simulink model "sunsensor_validity_and_logic_test"  (R2018b)
settings: Solver=VariableStepAuto  StartTime=0.0  StopTime=10.0  RelTol=1e-3
undefined symbols (not defined in the file): simParams
libraries: CDH_command_lib x1, mode_select_lib x1, sunsensor_processing_lib x1
settings Model: Creator=Taylor  LastModifiedBy=Taylor

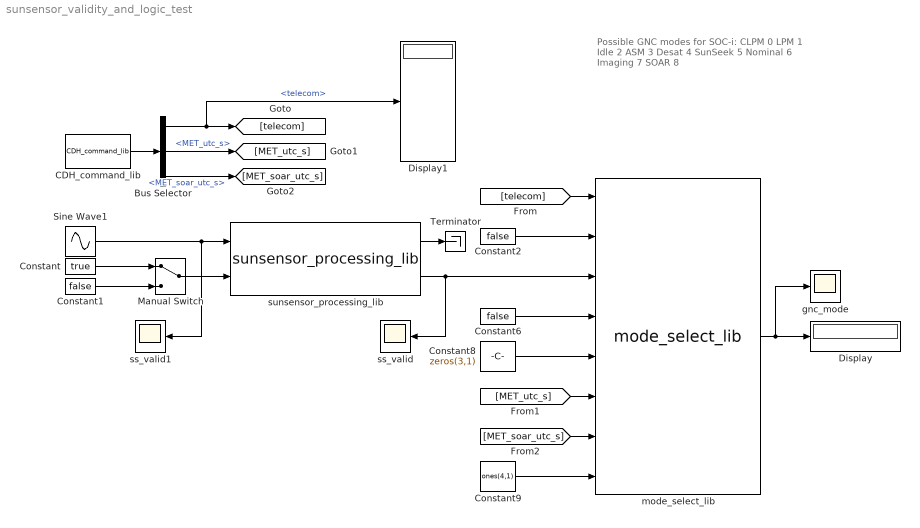
== system sunsensor_validity_and_logic_test ==
  note: Possible GNC modes for SOC-i:
      | CLPM 0
      | LPM 1
      | Idle 2
      | ASM 3
      | Desat 4
      | SunSeek 5
      | Nominal 6
      | Imaging 7
      | SOAR 8
  Bus Selector : BusSelector  OutputSignals=telecom,MET_utc_s,MET_soar_utc_s
  CDH_command_lib : CDH_command_lib/CDH_command_lib  target_lat_deg=47  target_lon_deg=-122  target_alt_m=44  override_autonomy=0  enable_pointing=on  force_clpm=off  force_lpm=off  enable_img=off  enable_soar=off  triad_override=off  MET_soar_utc_s=simParams.time.epoch_utc_s+2000  quat_soar_cmd=[1;0;0;0]
  Constant : Constant  Value=true
  Constant1 : Constant  Value=false
  Constant2 : Constant  Value=false
  Constant6 : Constant  Value=false
  Constant8 : Constant  Value=zeros(3,1)
  Constant9 : Constant  Value=ones(4,1)
  Display : Display
  Display1 : Display
  Manual Switch : ManualSwitch
  Sine Wave1 : Sin  Amplitude=[90 90]  Bias=[0 0]  Frequency=[1 1]  Phase=[0 0]  SampleTime=0
  Terminator : Terminator
  gnc_mode : Scope
  mode_select_lib : mode_select_lib/mode_select_lib  SystemSampleTime=-1
  ss_valid : Scope
  ss_valid1 : Scope
  sunsensor_processing_lib : sunsensor_processing_lib/sunsensor_processing_lib  SystemSampleTime=-1
  wires:
  Constant/1 -> Manual Switch/1
  Constant1/1 -> Manual Switch/2
  Sine Wave1/1 -> ss_valid1/1, sunsensor_processing_lib/1
  Bus Selector/2 -> [MET_utc_s]  "<MET_utc_s>"
  mode_select_lib/1 -> Display/1, gnc_mode/1
  sunsensor_processing_lib/2 -> ss_valid/1, mode_select_lib/3
  [telecom] -> mode_select_lib/1
  Constant6/1 -> mode_select_lib/4
  Constant8/1 -> mode_select_lib/5
  CDH_command_lib/1 -> Bus Selector/1
  Bus Selector/1 -> Display1/1, [telecom]  "<telecom>"
  [MET_utc_s] -> mode_select_lib/6
  Constant2/1 -> mode_select_lib/2
  [MET_soar_utc_s] -> mode_select_lib/7
  Bus Selector/3 -> [MET_soar_utc_s]  "<MET_soar_utc_s>"
  Manual Switch/1 -> sunsensor_processing_lib/2
  Constant9/1 -> mode_select_lib/8
  sunsensor_processing_lib/1 -> Terminator/1
